simulink model "distmodel_v4"  (R2020b)
settings: Solver=FixedStepAuto  StartTime=0.0  StopTime=t_sim  FixedStep=TimeStep  RelTol=1e-3
values from neighbouring files (symbols this model uses):
  alt = 300    [main_disturbances.m]    (also in simple_propagator.m)
  D = [x_th-x_cog;y_th-y_cog;z_th-z_cog]/1e3    [momentumstorage.m]
  inc = rad2deg(inc)    [main_disturbances.m]    (also in simple_propagator.m)
  nu = rad2deg(nu)    [main_disturbances.m]    (also in simple_propagator.m)
  RAAN = rad2deg(RAAN)    [main_disturbances.m]    (also in simple_propagator.m)
  w = find(volume(:,y,z) == 1)    [calc_torque_v1.m]    (also in main_disturbances.m = rad2deg(w); simple_propagator.m = rad2deg(w))
undefined symbols (not defined in the file or in its folder): date, ecc, IonSataero, km, s, sat, SNAP_CONST_a3H0, SNAP_CONST_earth_mag_dipole, SNAP_magnets, SNAP_starting_ECI2ECEF_dcm
libraries: vrlib x15, dspmathops x8, sharedtransform x7, aerolibutil x5, simulink_extras x2, simulink x2, aerolibtransform2 x2, aerolibconvert2 x1, sharedutil x1, aerolibcelestial x1
settings Model: Creator=colpari  LastModifiedBy=colpari

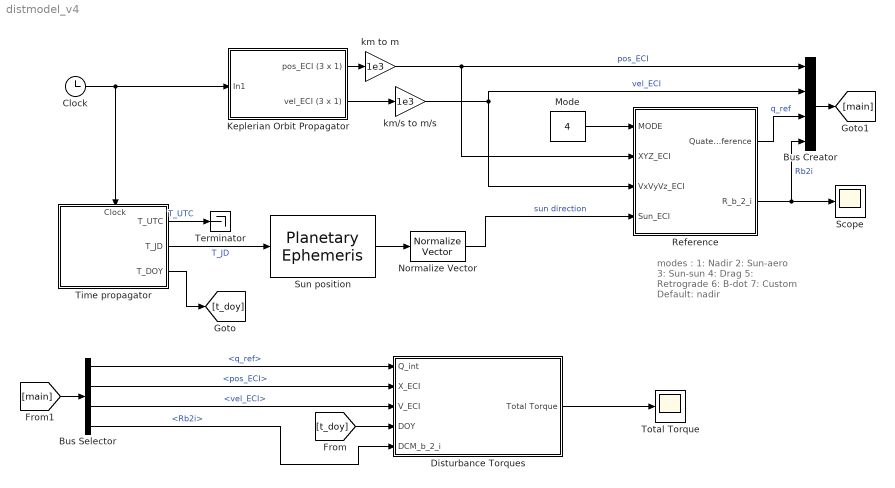
== system distmodel_v4 ==
  note: modes :
      | 1: Nadir
      | 2: Sun-aero
      | 3: Sun-sun
      | 4: Drag
      | 5: Retrograde
      | 6: B-dot
      | 7: Custom
      | Default: nadir
  Bus Creator : BusCreator  Inputs=4
  Bus Selector : BusSelector  OutputSignals=q_ref,pos_ECI,vel_ECI,Rb2i
  Clock : Clock
  "Disturbance Torques " : Subsystem
  Keplerian Orbit Propagator : Subsystem
  Mode : Constant  Value=4  OutDataTypeStr=int8
  Normalize Vector : vrlib/Utilities/Normalize Vector  maxzero=0
  Reference : Subsystem  TreatAsAtomicUnit=on
  Scope : Scope
  Sun position : aerolibcelestial/Planetary Ephemeris  kmflag=km,km/s  epochflag=Julian date  de=DE405  nCenter=Earth  nTarget=Sun  errorflag=Error  velflag=off
      settings: SourceProductBaseCode=AE
  Terminator : Terminator
  Time propagator : Subsystem
      settings: PortSchema="{\"entries\":[{\"content\":{\"sides\":[{\"content\":{\"connectorIds\":[]},\"type\":\"ConnectorPlacement.EquallySpacedRectSide\",\"uuid\":\"7ef5eb6e-74fd-40ed-a8ee-9d1a69b44829\"},{\"content\":{\"connectorIds\":[\"Out1\",\"Out2\",\"Out3\"],\"side\":\"RIGHT\"},\"type\":\"ConnectorPlacement.EquallySpacedRectSide\",\"uuid\":\"c2943143-c830-4f44-8257-0a7a59c653c3\"},{\"content\":{\"connectorIds\":[\"In1\"],\"side\":\"TOP\"},\"type\":\"ConnectorPlacement.EquallySpacedRectSide\",\"uuid\":\"75bbb385-8914-422a-90cf-596677817ce3\"},{\"content\":{\"connectorIds\":[],\"side\":\"HIDDEN\"},\"type\":\"ConnectorPlacement.EquallySpacedRectSide\",\"uuid\":\"39fbcd54-eaf8-409f-b881-9096903d4fff\"}]},\"type\":\"ConnectorPlacement.EquallySpacedConnector\",\"uuid\":\"f15d11f7-34b5-45ba-967f-26d924bb8ffd\"}],\"packageUris\":[\"http://schema.mathworks.com/mf0/Connector/R2020b\"],\"version\":\"1.0\"}"
  Total Torque : Scope
  km to m : Gain  Gain=1e3
  km/s to m/s : Gain  Gain=1e3
  wires:
  [t_doy] -> "Disturbance Torques "/4(DOY)
  "Disturbance Torques "/1("Total Torque ") -> Total Torque/1
  Bus Selector/3 -> "Disturbance Torques "/3(V_ECI)  "<vel_ECI>"
  Bus Selector/2 -> "Disturbance Torques "/2(X_ECI)  "<pos_ECI>"
  Clock/1 -> Keplerian Orbit Propagator/1(In1), Time propagator/1(Clock)
  Keplerian Orbit Propagator/1(pos_ECI (3 x 1)) -> km to m/1
  Keplerian Orbit Propagator/2(vel_ECI (3 x 1)) -> km/s to m/s/1
  Sun position/1 -> Normalize Vector/1
  Normalize Vector/1 -> Reference/4(Sun_ECI)  "sun direction"
  Time propagator/2(T_JD) -> Sun position/1  "T_JD"
  Reference/1(Quaternion Reference) -> Bus Creator/3  "q_ref"
  Time propagator/3(T_DOY) -> [t_doy]
  Bus Creator/1 -> [main]
  Time propagator/1(T_UTC) -> Terminator/1  "T_UTC"
  [main] -> Bus Selector/1
  km to m/1 -> Bus Creator/1, Reference/2(XYZ_ECI)  "pos_ECI"
  km/s to m/s/1 -> Bus Creator/2, Reference/3(VxVyVz_ECI)  "vel_ECI"
  Bus Selector/1 -> "Disturbance Torques "/1("Q_int ")  "<q_ref>"
  Reference/2(R_b_2_i) -> Bus Creator/4, Scope/1  "Rb2i"
  Bus Selector/4 -> "Disturbance Torques "/5(DCM_b_2_i)  "<Rb2i>"
  Mode/1 -> Reference/1(MODE)

== system distmodel_v4/Disturbance Torques  ==
  "Q_int " : Inport
  X_ECI : Inport  Port=2
  V_ECI : Inport  Port=3
  DOY : Inport  Port=4
  DCM_b_2_i : Inport  Port=5
  2 dist torques : Scope  NumInputPorts=2
  Add1 : Sum
  Aerodynamic Model : Subsystem
  Gravity Gradient Model : Subsystem
  Magnets : Subsystem  Commented=on
  Transpose1 : Math  Operator=transpose  SaturateOnIntegerOverflow=on
  "Total Torque " : Outport
  wires:
  Add1/1 -> "Total Torque "/1
  V_ECI/1 -> Aerodynamic Model/1(Velocity  (V) [m/s])
  X_ECI/1 -> Aerodynamic Model/2(Position (X) [m]), Gravity Gradient Model/1("Position (X) [m] ")
  Aerodynamic Model/2(Aero. Torque [N.m]1) -> 2 dist torques/1, Add1/1
  Gravity Gradient Model/1(Gravity Gradient [N.m]) -> 2 dist torques/2, Add1/2
  DCM_b_2_i/1 -> Transpose1/1
  Transpose1/1 -> Aerodynamic Model/3(Attitude (DCM_i2b)), Gravity Gradient Model/2(Attitude (DCMi2b))
  "Q_int "/1 -> Aerodynamic Model/4(Qref)

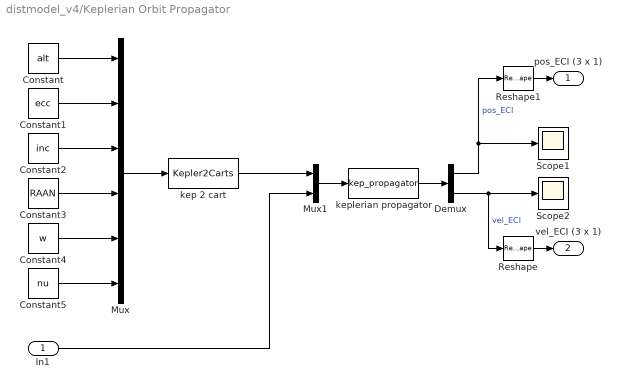
== system distmodel_v4/Keplerian Orbit Propagator ==
  In1 : Inport
  Constant : Constant  Value=alt
  Constant1 : Constant  Value=ecc
  Constant2 : Constant  Value=inc
  Constant3 : Constant  Value=RAAN
  Constant4 : Constant  Value=w
  Constant5 : Constant  Value=nu
  Demux : Demux  Outputs=2
  Mux : Mux  Inputs=6
  Mux1 : Mux  Inputs=2
  Reshape : Reshape  OutputDimensionality=Column vector (2-D)  OutputDimensions=[1,3]
  Reshape1 : Reshape  OutputDimensionality=Column vector (2-D)
  Scope1 : Scope
  Scope2 : Scope
  kep 2 cart : MATLABFcn  MATLABFcn=Kepler2Carts
  keplerian propagator : MATLABFcn  MATLABFcn=kep_propagator
  pos_ECI (3 x 1) : Outport
  vel_ECI (3 x 1) : Outport  Port=2
  wires:
  Mux/1 -> kep 2 cart/1
  Constant5/1 -> Mux/6
  Constant2/1 -> Mux/3
  kep 2 cart/1 -> Mux1/1
  Demux/2 -> Reshape/1, Scope2/1  "vel_ECI"
  Constant3/1 -> Mux/4
  Demux/1 -> Reshape1/1, Scope1/1  "pos_ECI"
  Constant4/1 -> Mux/5
  keplerian propagator/1 -> Demux/1
  Mux1/1 -> keplerian propagator/1
  Constant/1 -> Mux/1
  Constant1/1 -> Mux/2
  In1/1 -> Mux1/2
  Reshape/1 -> vel_ECI (3 x 1)/1
  Reshape1/1 -> pos_ECI (3 x 1)/1

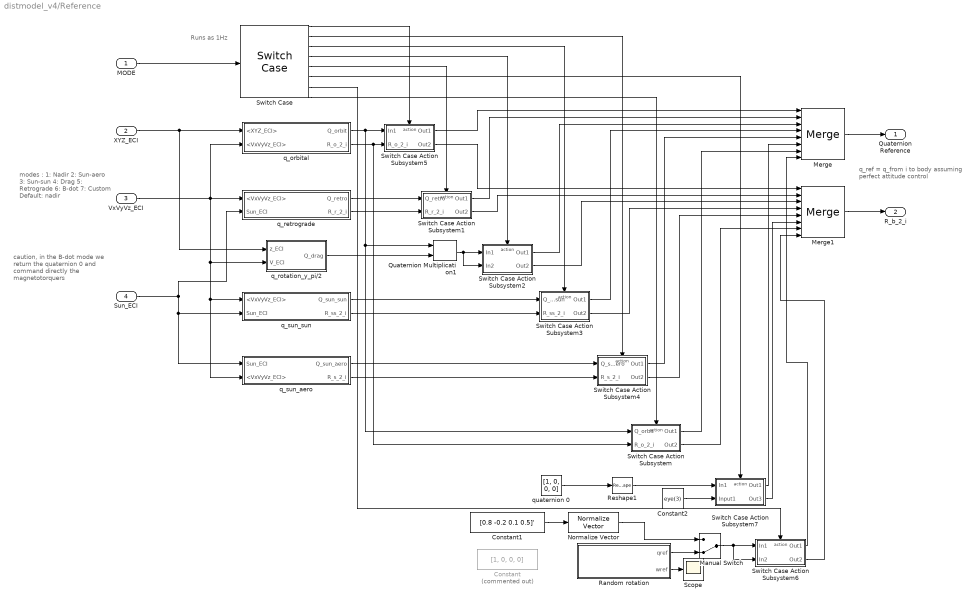
== system distmodel_v4/Reference ==
  note: caution, in the B-dot mode we return the quaternion 0 and command directly the magnetotorquers
  note: modes :
      | 1: Nadir
      | 2: Sun-aero
      | 3: Sun-sun
      | 4: Drag
      | 5: Retrograde
      | 6: B-dot
      | 7: Custom
      | Default: nadir
  note: Runs as 1Hz
  note: q_ref  = q_from i to body
      | assuming perfect attitude control
  MODE : Inport  OutMin=1  OutMax=100  OutDataTypeStr=int8
  XYZ_ECI : Inport  Port=2
  VxVyVz_ECI : Inport  Port=3
  Sun_ECI : Inport  Port=4
  Constant : Constant  Commented=on  Value=[1, 0, 0, 0]
  Constant1 : Constant  Value=[0.8 -0.2 0.1 0.5]'
  Constant2 : Constant  Value=eye(3)
  Manual Switch : ManualSwitch  CurrentSetting=0
  Merge : Merge  Inputs=8
  Merge1 : Merge  Inputs=8
  Normalize Vector : vrlib/Utilities/Normalize Vector  maxzero=0
  Quaternion Multiplication1 : aerolibutil/Quaternion Multiplication
  Random rotation : Subsystem
  Reshape1 : Reshape  OutputDimensionality=Column vector (2-D)
  Scope : Scope
  Switch Case : SwitchCase  CaseConditions={1, 2, 3, 4, 5, 6, 7}
  Switch Case Action Subsystem : Subsystem  TreatAsAtomicUnit=on
  Switch Case Action Subsystem1 : Subsystem  TreatAsAtomicUnit=on
  Switch Case Action Subsystem2 : Subsystem  TreatAsAtomicUnit=on
  Switch Case Action Subsystem3 : Subsystem  TreatAsAtomicUnit=on
  Switch Case Action Subsystem4 : Subsystem  TreatAsAtomicUnit=on
  Switch Case Action Subsystem5 : Subsystem  TreatAsAtomicUnit=on
  Switch Case Action Subsystem6 : Subsystem  TreatAsAtomicUnit=on
  Switch Case Action Subsystem7 : Subsystem  TreatAsAtomicUnit=on
  q_orbital : Subsystem
  q_retrograde : Subsystem
  q_rotation_y_pi/2 : Subsystem
  q_sun_aero : Subsystem
  q_sun_sun : Subsystem
  quaternion 0 : Constant  Value=[1, 0, 0, 0]
  Quaternion Reference : Outport  VectorParamsAs1DForOutWhenUnconnected=off
  R_b_2_i : Outport  Port=2
  wires:
  q_sun_sun/1(Q_sun_sun) -> Switch Case Action Subsystem3/1(Q_sun_sun)
  Sun_ECI/1 -> q_retrograde/2(Sun_ECI), q_sun_aero/1(Sun_ECI), q_sun_sun/2(Sun_ECI)
  MODE/1 -> Switch Case/1
  q_rotation_y_pi/2/1(Q_drag) -> Quaternion Multiplication1/2
  Switch Case/3 -> Switch Case Action Subsystem3/Action
  q_sun_aero/1(Q_sun_aero) -> Switch Case Action Subsystem4/1(Q_sun_aero)
  Merge/1 -> Quaternion Reference/1
  XYZ_ECI/1 -> q_orbital/1(<XYZ_ECI>), q_rotation_y_pi/2/1(z_ECI)
  Switch Case/5 -> Switch Case Action Subsystem1/Action
  Switch Case/4 -> Switch Case Action Subsystem2/Action
  quaternion 0/1 -> Reshape1/1
  VxVyVz_ECI/1 -> q_orbital/2(<VxVyVz_ECI>), q_retrograde/1(<VxVyVz_ECI>), q_sun_aero/2(<VxVyVz_ECI>), q_sun_sun/1(<VxVyVz_ECI>), q_rotation_y_pi/2/2(V_ECI)
  Switch Case/2 -> Switch Case Action Subsystem4/Action
  Quaternion Multiplication1/1 -> Switch Case Action Subsystem2/2(In2), Switch Case Action Subsystem2/1(In1)
  q_orbital/1(Q_orbit) -> Switch Case Action Subsystem5/1(In1), Quaternion Multiplication1/1, Switch Case Action Subsystem/1(Q_orbit)
  Switch Case/6 -> Switch Case Action Subsystem7/Action
  q_retrograde/1(Q_retro) -> Switch Case Action Subsystem1/1(Q_retro)
  Reshape1/1 -> Switch Case Action Subsystem7/1(In1)
  Merge1/1 -> R_b_2_i/1
  Switch Case Action Subsystem5/1(Out1) -> Merge/1
  Switch Case Action Subsystem5/2(Out2) -> Merge1/1
  Switch Case Action Subsystem1/1(Out1) -> Merge/2
  Switch Case Action Subsystem1/2(Out2) -> Merge1/2
  Switch Case Action Subsystem2/1(Out1) -> Merge/3
  Switch Case Action Subsystem2/2(Out2) -> Merge1/3
  Switch Case Action Subsystem3/1(Out1) -> Merge/4
  Switch Case Action Subsystem3/2(Out2) -> Merge1/4
  Switch Case Action Subsystem4/1(Out1) -> Merge/5
  Switch Case Action Subsystem4/2(Out2) -> Merge1/5
  Switch Case Action Subsystem/1(Out1) -> Merge/7
  Switch Case Action Subsystem/2(Out2) -> Merge1/7
  Switch Case Action Subsystem7/1(Out1) -> Merge/6
  Switch Case Action Subsystem7/2(Out3) -> Merge1/6
  Switch Case/1 -> Switch Case Action Subsystem5/Action
  Switch Case/8 -> Switch Case Action Subsystem/Action
  Switch Case/7 -> Switch Case Action Subsystem6/Action
  Switch Case Action Subsystem6/1(Out1) -> Merge/8
  Switch Case Action Subsystem6/2(Out2) -> Merge1/8
  Constant1/1 -> Normalize Vector/1
  Normalize Vector/1 -> Manual Switch/1
  Manual Switch/1 -> Switch Case Action Subsystem6/2(In2), Switch Case Action Subsystem6/1(In1)
  q_orbital/2(R_o_2_i) -> Switch Case Action Subsystem/2(R_o_2_i), Switch Case Action Subsystem5/2(R_o_2_i)
  q_sun_aero/2(R_s_2_i) -> Switch Case Action Subsystem4/2(R_s_2_i)
  q_sun_sun/2(R_ss_2_i) -> Switch Case Action Subsystem3/2(R_ss_2_i)
  q_retrograde/2(R_r_2_i) -> Switch Case Action Subsystem1/2(R_r_2_i)
  Constant2/1 -> Switch Case Action Subsystem7/2(Input1)
  Random rotation/1(qref) -> Manual Switch/2
  Random rotation/2(wref) -> Scope/1

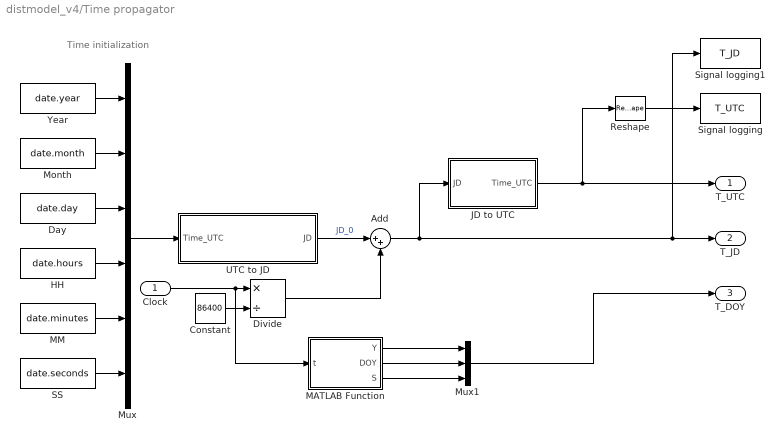
== system distmodel_v4/Time propagator ==
  note: Time initialization
  Clock : Inport
  Add : Sum  Inputs=|++
  Constant : Constant  Value=86400
  Day : Constant  Value=date.day
  Divide : Product  Inputs=*/
  HH : Constant  Value=date.hours
  JD to UTC : MATLAB Function  TreatAsAtomicUnit=on
  MATLAB Function : MATLAB Function  TreatAsAtomicUnit=on
  MM : Constant  Value=date.minutes
  Month : Constant  Value=date.month
  Mux : Mux  Inputs=6
  Mux1 : Mux  Inputs=3
  Reshape : Reshape
  SS : Constant  Value=date.seconds
  Signal logging : ToWorkspace  VariableName=T_UTC  SaveFormat=Timeseries  SampleTime=1
      settings: Save2DSignal=2-D array (concatenate along first dimension)
  Signal logging1 : ToWorkspace  VariableName=T_JD  SaveFormat=Timeseries  SampleTime=1
      settings: Save2DSignal=2-D array (concatenate along first dimension)
  UTC to JD : MATLAB Function  TreatAsAtomicUnit=on
  Year : Constant  Value=date.year
  T_UTC : Outport  VectorParamsAs1DForOutWhenUnconnected=off
  T_JD : Outport  Port=2  VectorParamsAs1DForOutWhenUnconnected=off
  T_DOY : Outport  Port=3
  wires:
  UTC to JD/1(JD) -> Add/1  "JD_0"
  Clock/1 -> MATLAB Function/1(t), Divide/1
  Constant/1 -> Divide/2
  JD to UTC/1(Time_UTC) -> T_UTC/1, Reshape/1
  Divide/1 -> Add/2
  Mux/1 -> UTC to JD/1(Time_UTC)
  Day/1 -> Mux/3
  Month/1 -> Mux/2
  Year/1 -> Mux/1
  HH/1 -> Mux/4
  MM/1 -> Mux/5
  SS/1 -> Mux/6
  Reshape/1 -> Signal logging/1
  Add/1 -> Signal logging1/1, T_JD/1, JD to UTC/1(JD)
  MATLAB Function/1(Y) -> Mux1/1
  MATLAB Function/2(DOY) -> Mux1/2
  MATLAB Function/3(S) -> Mux1/3
  Mux1/1 -> T_DOY/1

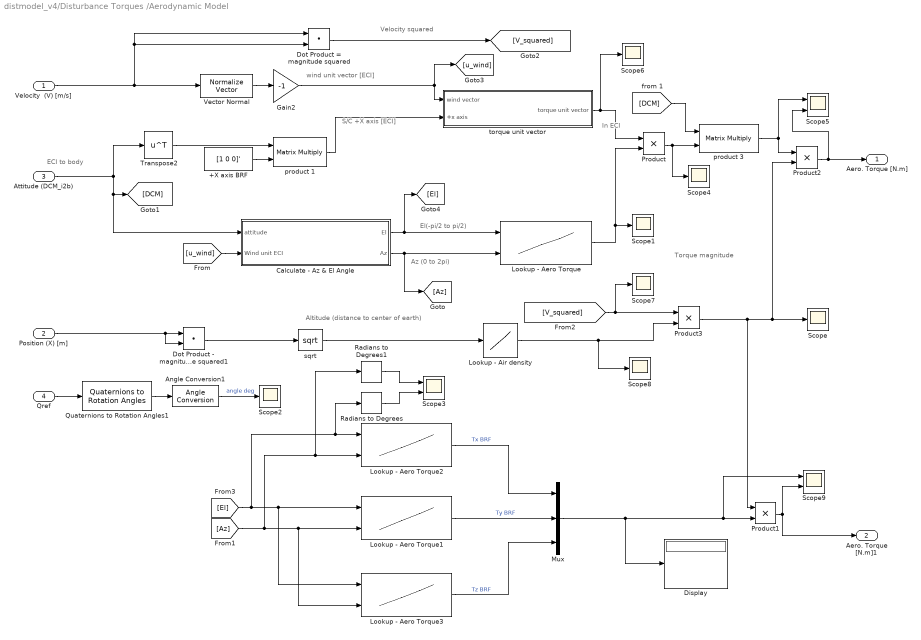
== system distmodel_v4/Disturbance Torques /Aerodynamic Model ==
  note: Az (0 to 2pi)
  note: wind unit vector [ECI]
  note: Torque magnitude
  note: S/C +X axis [ECI]
  note: In ECI
  note: ECI to body
  note: Velocity squared
  note: El(-pi/2 to pi/2)
  note: Altitude (distance to center of earth)
  Velocity  (V) [m/s] : Inport
  Position (X) [m] : Inport  Port=2
  Attitude (DCM_i2b) : Inport  Port=3
  Qref : Inport  Port=4
  +X axis BRF : Constant  Value=[1 0 0]'
  Angle Conversion1 : aerolibconvert2/Angle Conversion  IU=rad  OU=deg
  Calculate - Az & El Angle : Subsystem
  Display : Display
  Dot Product - magnitude squared1 : DotProduct  InputSameDT=on  OutDataTypeStr=Inherit: Inherit via internal rule
  Dot Product = magnitude squared : DotProduct  InputSameDT=on  OutDataTypeStr=Inherit: Inherit via internal rule
  Gain2 : Gain  Gain=-1
  Lookup - Aero Torque : Lookup2D  RowIndex=IonSataero.Az  ColumnIndex=IonSataero.El  Table=IonSataero.T
  Lookup - Aero Torque1 : Lookup2D  RowIndex=IonSataero.Az  ColumnIndex=IonSataero.El  Table=IonSataero.Ty
  Lookup - Aero Torque2 : Lookup2D  RowIndex=IonSataero.Az  ColumnIndex=IonSataero.El  Table=IonSataero.Tx
  Lookup - Aero Torque3 : Lookup2D  RowIndex=IonSataero.Az  ColumnIndex=IonSataero.El  Table=IonSataero.Tz
  Lookup - Air density : Lookup  InputValues=IonSataero.alt_range*1000 + 6378100  Table=IonSataero.av_density_vs_alt
  Mux : Mux  Inputs=3
  Product{,1..3} (4 alike) : Product  RndMeth=Zero
  Quaternions to Rotation Angles1 : sharedtransform/Quaternions to Rotation Angles  rotationOrder=ZYX  aMode=aMode
      settings: SourceProductBaseCode=AE,PW,MT,UV,VE,VP
  Radians to Degrees : simulink_extras/Transformations/Radians to Degrees
  Radians to Degrees1 : simulink_extras/Transformations/Radians to Degrees
  Scope{,1..2,4,6..8} (7 alike) : Scope
  Scope3 : Scope  NumInputPorts=2
  Scope5 : Scope  NumInputPorts=2
  Scope9 : Scope  NumInputPorts=2
  Transpose2 : Math  Operator=transpose  SignedPower=on  SaturateOnIntegerOverflow=on
  Vector Normal : vrlib/Utilities/Normalize Vector  maxzero=0
  product 1 : Product  Multiplication=Matrix(*)  RndMeth=Zero
  product 3 : Product  Multiplication=Matrix(*)  RndMeth=Zero
  sqrt : Math  Operator=sqrt  SignedPower=on  SaturateOnIntegerOverflow=on
  torque unit vector : Subsystem
  Aero. Torque [N.m] : Outport
  Aero. Torque [N.m]1 : Outport  Port=2
  wires:
  Dot Product = magnitude squared/1 -> [V_squared]
  Vector Normal/1 -> Gain2/1
  Gain2/1 -> [u_wind], torque unit vector/1(wind vector)
  product 1/1 -> torque unit vector/2(+x axis)
  torque unit vector/1(torque unit vector) -> Scope6/1, Product/1
  Lookup - Aero Torque/1 -> Scope1/1, Product/2
  [DCM] -> product 3/1
  +X axis BRF/1 -> product 1/2
  Product/1 -> Scope4/1, product 3/2
  Transpose2/1 -> product 1/1
  Attitude (DCM_i2b)/1 -> Calculate - Az & El Angle/1(attitude), [DCM], Transpose2/1
  Position (X) [m]/1 -> Dot Product - magnitude squared1/1, Dot Product - magnitude squared1/2
  Dot Product - magnitude squared1/1 -> sqrt/1
  sqrt/1 -> Lookup - Air density/1
  Lookup - Air density/1 -> Scope8/1, Product3/2
  [V_squared] -> Scope7/1, Product3/1
  Product2/1 -> Scope5/2, Aero. Torque [N.m]/1
  product 3/1 -> Scope5/1, Product2/1
  Velocity  (V) [m/s]/1 -> Vector Normal/1, Dot Product = magnitude squared/2, Dot Product = magnitude squared/1
  Radians to Degrees1/1 -> Scope3/1
  Radians to Degrees/1 -> Scope3/2
  Qref/1 -> Quaternions to Rotation Angles1/1
  Quaternions to Rotation Angles1/1 -> Angle Conversion1/1
  Angle Conversion1/1 -> Scope2/1  "angle deg"
  [u_wind] -> Calculate - Az & El Angle/2(Wind unit ECI)
  Calculate - Az & El Angle/2(Az) -> [Az], Lookup - Aero Torque/2
  Calculate - Az & El Angle/1(El) -> [El], Lookup - Aero Torque/1
  [El] -> Radians to Degrees/1, Lookup - Aero Torque2/1, Lookup - Aero Torque3/1, Lookup - Aero Torque1/1
  [Az] -> Radians to Degrees1/1, Lookup - Aero Torque2/2, Lookup - Aero Torque3/2, Lookup - Aero Torque1/2
  Lookup - Aero Torque1/1 -> Mux/2  "Ty BRF"
  Lookup - Aero Torque2/1 -> Mux/1  "Tx BRF"
  Lookup - Aero Torque3/1 -> Mux/3  "Tz BRF"
  Mux/1 -> Display/1, Product1/2, Scope9/1
  Product3/1 -> Product1/1, Scope/1, Product2/2
  Product1/1 -> Aero. Torque [N.m]1/1, Scope9/2

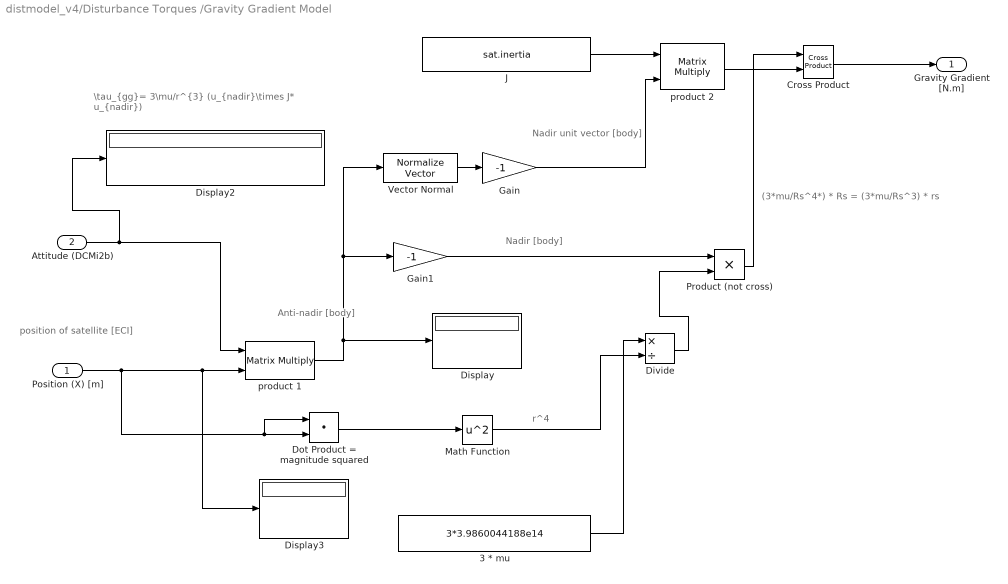
== system distmodel_v4/Disturbance Torques /Gravity Gradient Model ==
  note: \tau_{gg}= 3\mu/r^{3} (u_{nadir}\times J* u_{nadir})
  note: (3*mu/Rs^4*) * Rs = (3*mu/Rs^3) * rs
  note: Nadir [body]
  note: position of satellite [ECI]
  note: Nadir unit vector
      | [body]
  note: Anti-nadir [body]
  note: r^4
  "Position (X) [m] " : Inport
  Attitude (DCMi2b) : Inport  Port=2
  3 * mu : Constant  Value=3*3.9860044188e14
  Cross Product : vrlib/Utilities/Cross Product
  Display : Display
  Display2 : Display
  Display3 : Display
  Divide : Product  Inputs=*/
  Dot Product = magnitude squared : DotProduct  InputSameDT=on  OutDataTypeStr=Inherit: Inherit via internal rule
  Gain : Gain  Gain=-1
  Gain1 : Gain  Gain=-1
  J : Constant  Value=sat.inertia
  Math Function : Math  Operator=square  SignedPower=on  SaturateOnIntegerOverflow=on
  Product (not cross) : Product  RndMeth=Zero
  Vector Normal : vrlib/Utilities/Normalize Vector  maxzero=0
  product 1 : Product  Multiplication=Matrix(*)  RndMeth=Zero
  product 2 : Product  Multiplication=Matrix(*)  RndMeth=Zero
  Gravity Gradient [N.m] : Outport
  wires:
  Product (not cross)/1 -> Cross Product/1
  Divide/1 -> Product (not cross)/2
  3 * mu/1 -> Divide/1
  Math Function/1 -> Divide/2
  Vector Normal/1 -> Gain/1
  Cross Product/1 -> Gravity Gradient [N.m]/1
  Dot Product = magnitude squared/1 -> Math Function/1
  Gain/1 -> product 2/2
  product 2/1 -> Cross Product/2
  J/1 -> product 2/1
  Attitude (DCMi2b)/1 -> Display2/1, product 1/1
  product 1/1 -> Vector Normal/1, Gain1/1, Display/1
  Gain1/1 -> Product (not cross)/1
  "Position (X) [m] "/1 -> product 1/2, Display3/1, Dot Product = magnitude squared/2, Dot Product = magnitude squared/1

== system distmodel_v4/Disturbance Torques /Magnets ==
  note: T = m X B
  note: B_earth [body]
  note: ECI to Body
  Position (X) : Inport
  Attitude (DCM) : Inport  Port=2
  Cross Product : vrlib/Utilities/Cross Product
  Eearth L-Shell Magnetic Model : Subsystem
  Product : Product  Multiplication=Matrix(*)  RndMeth=Zero
  Transpose : Math  Operator=transpose  SignedPower=on  SaturateOnIntegerOverflow=on
  constant : Constant  Value=SNAP_magnets
  MagneticTorque (N.m) : Outport
  B (Tesla) [ECI] : Outport  Port=2
  wires:
  Position (X)/1 -> Eearth L-Shell Magnetic Model/1(Position in ECI)
  Product/1 -> Cross Product/2
  Cross Product/1 -> MagneticTorque (N.m)/1
  constant/1 -> Cross Product/1
  Attitude (DCM)/1 -> Product/1
  Eearth L-Shell Magnetic Model/1(B (Tesla) in ECI) -> Transpose/1, B (Tesla) [ECI]/1
  Transpose/1 -> Product/2

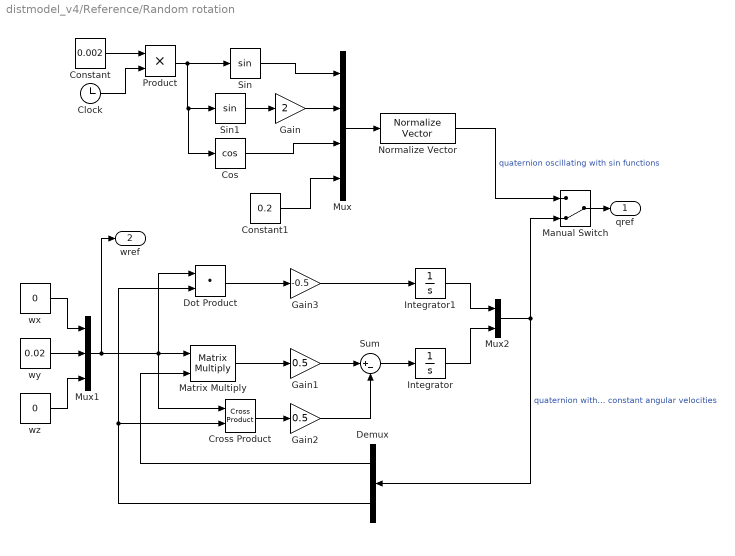
== system distmodel_v4/Reference/Random rotation ==
  Clock : Clock
      settings: Decimation=TimeStep
  Constant : Constant  Value=0.002
  Constant1 : Constant  Value=0.2
  Cos : Trigonometry  Operator=cos
  Cross Product : vrlib/Utilities/Cross Product
  Demux : Demux  Outputs=[1;3]
  Dot Product : DotProduct  InputSameDT=on  OutDataTypeStr=Inherit: Inherit via internal rule
  Gain : Gain  Gain=2
  Gain1 : Gain  Gain=0.5
  Gain2 : Gain  Gain=0.5
  Gain3 : Gain  Gain=-0.5
  Integrator : Integrator  InitialCondition=[0;0;0]
  Integrator1 : Integrator  InitialCondition=1
  Manual Switch : ManualSwitch  CurrentSetting=0
  Matrix Multiply : Product  Multiplication=Matrix(*)
  Mux : Mux
  Mux1 : Mux  Inputs=3
  Mux2 : Mux  Inputs=[1;3]
  Normalize Vector : vrlib/Utilities/Normalize Vector  maxzero=0
  Product : Product
  Sin : Trigonometry
  Sin1 : Trigonometry
  Sum : Sum  Inputs=|+-
  wx : Constant  Value=0
  wy : Constant  Value=0.02
  wz : Constant  Value=0
  qref : Outport
  wref : Outport  Port=2
  wires:
  Mux/1 -> Normalize Vector/1
  Normalize Vector/1 -> Manual Switch/1  "quaternion oscillating with sin functions"
  Constant/1 -> Product/1
  Clock/1 -> Product/2
  Product/1 -> Cos/1, Sin1/1, Sin/1
  Sin/1 -> Mux/1
  Sin1/1 -> Gain/1
  Gain/1 -> Mux/2
  Cos/1 -> Mux/3
  Constant1/1 -> Mux/4
  Manual Switch/1 -> qref/1
  wx/1 -> Mux1/1
  wy/1 -> Mux1/2
  wz/1 -> Mux1/3
  Mux1/1 -> wref/1, Dot Product/1, Cross Product/1, Matrix Multiply/1
  Matrix Multiply/1 -> Gain1/1
  Gain1/1 -> Sum/1
  Sum/1 -> Integrator/1
  Integrator/1 -> Mux2/2
  Mux2/1 -> Demux/1, Manual Switch/2  "quaternion with constant angular velocities"
  Demux/1 -> Matrix Multiply/2
  Cross Product/1 -> Gain2/1
  Gain2/1 -> Sum/2
  Dot Product/1 -> Gain3/1
  Gain3/1 -> Integrator1/1
  Integrator1/1 -> Mux2/1
  Demux/2 -> Cross Product/2, Dot Product/2

== system distmodel_v4/Reference/Switch Case Action Subsystem ==
  Q_orbit : Inport
  R_o_2_i : Inport  Port=2
  Action Port : ActionPort  ActionPortLabel=default:
  Out1 : Outport  VectorParamsAs1DForOutWhenUnconnected=off
  Out2 : Outport  Port=2  VectorParamsAs1DForOutWhenUnconnected=off
  wires:
  Q_orbit/1 -> Out1/1
  R_o_2_i/1 -> Out2/1

== system distmodel_v4/Reference/Switch Case Action Subsystem1 ==
  Q_retro : Inport
  R_r_2_i : Inport  Port=2
  Action Port : ActionPort  ActionPortLabel=case [ 5 ]:
  Out1 : Outport  VectorParamsAs1DForOutWhenUnconnected=off
  Out2 : Outport  Port=2  VectorParamsAs1DForOutWhenUnconnected=off
  wires:
  Q_retro/1 -> Out1/1
  R_r_2_i/1 -> Out2/1

== system distmodel_v4/Reference/Switch Case Action Subsystem2 ==
  In1 : Inport
  In2 : Inport  Port=2
  Action Port : ActionPort  ActionPortLabel=case [ 4 ]:
  Quaternions to Direction Cosine Matrix : sharedtransform/Quaternions to  Direction Cosine Matrix  aMode=aMode
      settings: SourceProductBaseCode=AE,PW,MT,UV,VE,VP
  Out1 : Outport  VectorParamsAs1DForOutWhenUnconnected=off
  Out2 : Outport  Port=2  VectorParamsAs1DForOutWhenUnconnected=off
  wires:
  In1/1 -> Out1/1
  In2/1 -> Quaternions to Direction Cosine Matrix/1
  Quaternions to Direction Cosine Matrix/1 -> Out2/1

== system distmodel_v4/Reference/Switch Case Action Subsystem3 ==
  Q_sun_sun : Inport
  R_ss_2_i : Inport  Port=2
  Action Port : ActionPort  ActionPortLabel=case [ 3 ]:
  Out1 : Outport  VectorParamsAs1DForOutWhenUnconnected=off
  Out2 : Outport  Port=2  VectorParamsAs1DForOutWhenUnconnected=off
  wires:
  Q_sun_sun/1 -> Out1/1
  R_ss_2_i/1 -> Out2/1

== system distmodel_v4/Reference/Switch Case Action Subsystem4 ==
  Q_sun_aero : Inport
  R_s_2_i : Inport  Port=2
  Action Port : ActionPort  ActionPortLabel=case [ 2 ]:
  Out1 : Outport  VectorParamsAs1DForOutWhenUnconnected=off
  Out2 : Outport  Port=2  VectorParamsAs1DForOutWhenUnconnected=off
  wires:
  Q_sun_aero/1 -> Out1/1
  R_s_2_i/1 -> Out2/1

== system distmodel_v4/Reference/Switch Case Action Subsystem5 ==
  In1 : Inport
  R_o_2_i : Inport  Port=2
  Action Port : ActionPort  ActionPortLabel=case [ 1 ]:
  Out1 : Outport  VectorParamsAs1DForOutWhenUnconnected=off
  Out2 : Outport  Port=2  VectorParamsAs1DForOutWhenUnconnected=off
  wires:
  In1/1 -> Out1/1
  R_o_2_i/1 -> Out2/1

== system distmodel_v4/Reference/Switch Case Action Subsystem6 ==
  In1 : Inport
  In2 : Inport  Port=2
  Action Port : ActionPort  ActionPortLabel=case [ 7 ]:
  Quaternions to Direction Cosine Matrix : sharedtransform/Quaternions to  Direction Cosine Matrix  aMode=aMode
      settings: SourceProductBaseCode=AE,PW,MT,UV,VE,VP
  Out1 : Outport  VectorParamsAs1DForOutWhenUnconnected=off
  Out2 : Outport  Port=2  VectorParamsAs1DForOutWhenUnconnected=off
  wires:
  In1/1 -> Out1/1
  In2/1 -> Quaternions to Direction Cosine Matrix/1
  Quaternions to Direction Cosine Matrix/1 -> Out2/1

== system distmodel_v4/Reference/Switch Case Action Subsystem7 ==
  In1 : Inport
  Input1 : Inport  Port=2
  Action Port : ActionPort  ActionPortLabel=case [ 6 ]:
  Out1 : Outport  VectorParamsAs1DForOutWhenUnconnected=off
  Out3 : Outport  Port=2  VectorParamsAs1DForOutWhenUnconnected=off
  wires:
  In1/1 -> Out1/1
  Input1/1 -> Out3/1

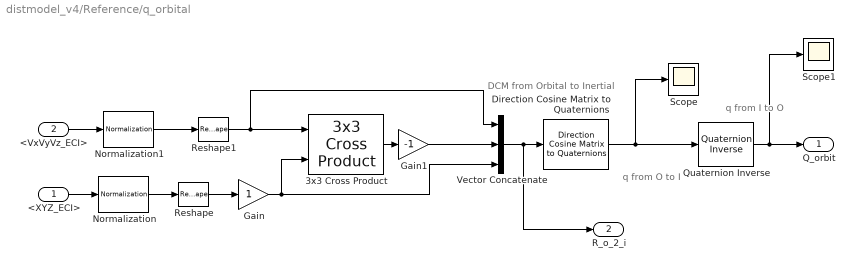
== system distmodel_v4/Reference/q_orbital ==
  note: DCM from Orbital to Inertial
  note: q from O to I
  note: q from I to O
  <XYZ_ECI> : Inport
  <VxVyVz_ECI> : Inport  Port=2
  3x3 Cross Product : sharedutil/3x3 Cross Product  aMode=aMode
      settings: SourceProductBaseCode=AE,PW,MT,UV,VE,VP
  Direction Cosine Matrix to Quaternions : sharedtransform/Direction Cosine Matrix  to Quaternions  aMode=0  action=None  tolerance=eps(2)
      settings: SourceProductBaseCode=AE,PW,MT,UV,VE,VP
  Gain : Gain
  Gain1 : Gain  Gain=-1
  Normalization : dspmathops/Normalization  NormType=2-norm  Bias=1e-10  NormOver=Each column  Dimension=1  roundingMode=Floor  overflowMode=off  accumDataTypeStr=Inherit: Same as product output  accumLastDataTypeStr=Inherit: Same as product output  outputDataTypeStr=Inherit: Same as product output  outputMin=[]  outputMax=[]  outputLastDataTypeStr=Inherit: Same as product output
  Normalization1 : dspmathops/Normalization  NormType=2-norm  Bias=1e-10  NormOver=Each column  Dimension=1  roundingMode=Floor  overflowMode=off  accumDataTypeStr=Inherit: Same as product output  accumLastDataTypeStr=Inherit: Same as product output  outputDataTypeStr=Inherit: Same as product output  outputMin=[]  outputMax=[]  outputLastDataTypeStr=Inherit: Same as product output
  Quaternion Inverse : aerolibutil/Quaternion Inverse
  Reshape : Reshape  OutputDimensionality=Column vector (2-D)
  Reshape1 : Reshape  OutputDimensionality=Column vector (2-D)
  Scope : Scope
  Scope1 : Scope
  Vector Concatenate : Concatenate  NumInputs=3  Mode=Multidimensional array  ConcatenateDimension=2
  Q_orbit : Outport  VectorParamsAs1DForOutWhenUnconnected=off
  R_o_2_i : Outport  Port=2  VectorParamsAs1DForOutWhenUnconnected=off
  wires:
  Normalization/1 -> Reshape/1
  Normalization1/1 -> Reshape1/1
  <VxVyVz_ECI>/1 -> Normalization1/1
  Reshape1/1 -> 3x3 Cross Product/1, Vector Concatenate/1
  <XYZ_ECI>/1 -> Normalization/1
  Reshape/1 -> Gain/1
  Gain/1 -> 3x3 Cross Product/2, Vector Concatenate/3
  Direction Cosine Matrix to Quaternions/1 -> Scope/1, Quaternion Inverse/1
  3x3 Cross Product/1 -> Gain1/1
  Gain1/1 -> Vector Concatenate/2
  Vector Concatenate/1 -> R_o_2_i/1, Direction Cosine Matrix to Quaternions/1
  Quaternion Inverse/1 -> Scope1/1, Q_orbit/1

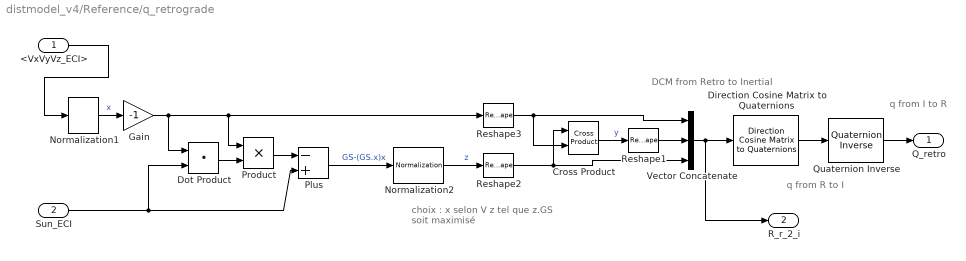
== system distmodel_v4/Reference/q_retrograde ==
  note: q from I to R
  note: q from R to I
  note: DCM from Retro to Inertial
  note: choix :
      | x selon V
      | z tel que z.GS soit maximisé
  <VxVyVz_ECI> : Inport
  Sun_ECI : Inport  Port=2
  Cross Product : vrlib/Utilities/Cross Product
  Direction Cosine Matrix to Quaternions : sharedtransform/Direction Cosine Matrix  to Quaternions  aMode=0  action=None  tolerance=eps(2)
      settings: SourceProductBaseCode=AE,PW,MT,UV,VE,VP
  Dot Product : DotProduct  InputSameDT=on  OutDataTypeStr=Inherit: Inherit via internal rule
  Gain : Gain  Gain=-1
  Normalization1 : dspmathops/Normalization  NormType=2-norm  Bias=1e-10  NormOver=Each column  Dimension=1  roundingMode=Floor  overflowMode=off  accumDataTypeStr=Inherit: Same as product output  accumLastDataTypeStr=Inherit: Same as product output  outputDataTypeStr=Inherit: Same as product output  outputMin=[]  outputMax=[]  outputLastDataTypeStr=Inherit: Same as product output
  Normalization2 : dspmathops/Normalization  NormType=2-norm  Bias=1e-10  NormOver=Each column  Dimension=1  roundingMode=Floor  overflowMode=off  accumDataTypeStr=Inherit: Same as product output  accumLastDataTypeStr=Inherit: Same as product output  outputDataTypeStr=Inherit: Same as product output  outputMin=[]  outputMax=[]  outputLastDataTypeStr=Inherit: Same as product output
  Plus : Sum  Inputs=-+
  Product : Product
  Quaternion Inverse : aerolibutil/Quaternion Inverse
  Reshape1 : Reshape  OutputDimensionality=Column vector (2-D)
  Reshape2 : Reshape  OutputDimensionality=Column vector (2-D)
  Reshape3 : Reshape  OutputDimensionality=Column vector (2-D)
  Vector Concatenate : Concatenate  NumInputs=3  Mode=Multidimensional array  ConcatenateDimension=2
  Q_retro : Outport  VectorParamsAs1DForOutWhenUnconnected=off
  R_r_2_i : Outport  Port=2  VectorParamsAs1DForOutWhenUnconnected=off
  wires:
  Quaternion Inverse/1 -> Q_retro/1
  Reshape2/1 -> Vector Concatenate/3, Cross Product/1
  Reshape3/1 -> Vector Concatenate/1, Cross Product/2
  Product/1 -> Plus/1
  Dot Product/1 -> Product/2
  Cross Product/1 -> Reshape1/1  "y"
  Normalization2/1 -> Reshape2/1  "z"
  Plus/1 -> Normalization2/1  "GS-(GS.x)x"
  Sun_ECI/1 -> Dot Product/2, Plus/2
  Vector Concatenate/1 -> R_r_2_i/1, Direction Cosine Matrix to Quaternions/1
  Direction Cosine Matrix to Quaternions/1 -> Quaternion Inverse/1
  Normalization1/1 -> Gain/1  "x"
  <VxVyVz_ECI>/1 -> Normalization1/1
  Reshape1/1 -> Vector Concatenate/2
  Gain/1 -> Dot Product/1, Product/1, Reshape3/1

== system distmodel_v4/Reference/q_rotation_y_pi//2 ==
  z_ECI : Inport
  V_ECI : Inport  Port=2
  Cross Product : vrlib/Utilities/Cross Product
  Product : Product
  Reshape1 : Reshape  OutputDimensionality=Column vector (2-D)
  Vector Concatenate1 : Concatenate  Mode=Multidimensional array
  cos pi/4 : Constant  Value=[sqrt(2)]
  sin pi/4 : Constant  Value=sqrt(2)
  Q_drag : Outport  VectorParamsAs1DForOutWhenUnconnected=off
  wires:
  cos pi/4/1 -> Vector Concatenate1/1
  Vector Concatenate1/1 -> Q_drag/1
  sin pi/4/1 -> Product/2
  z_ECI/1 -> Cross Product/1
  V_ECI/1 -> Cross Product/2
  Cross Product/1 -> Product/1  "y"
  Reshape1/1 -> Vector Concatenate1/2
  Product/1 -> Reshape1/1

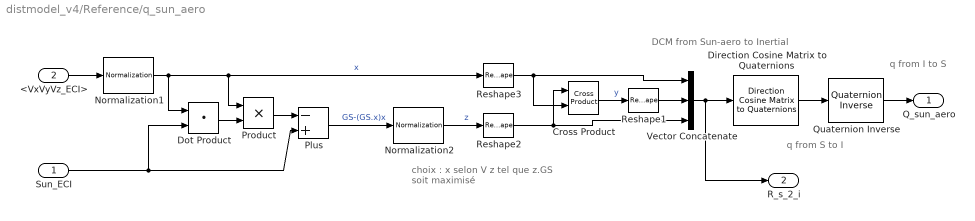
== system distmodel_v4/Reference/q_sun_aero ==
  note: q from I to S
  note: q from S to I
  note: DCM from Sun-aero to Inertial
  note: choix :
      | x selon V
      | z tel que z.GS soit maximisé
  Sun_ECI : Inport
  <VxVyVz_ECI> : Inport  Port=2
  Cross Product : vrlib/Utilities/Cross Product
  Direction Cosine Matrix to Quaternions : sharedtransform/Direction Cosine Matrix  to Quaternions  aMode=0  action=None  tolerance=eps(2)
      settings: SourceProductBaseCode=AE,PW,MT,UV,VE,VP
  Dot Product : DotProduct  InputSameDT=on  OutDataTypeStr=Inherit: Inherit via internal rule
  Normalization1 : dspmathops/Normalization  NormType=2-norm  Bias=1e-10  NormOver=Each column  Dimension=1  roundingMode=Floor  overflowMode=off  accumDataTypeStr=Inherit: Same as product output  accumLastDataTypeStr=Inherit: Same as product output  outputDataTypeStr=Inherit: Same as product output  outputMin=[]  outputMax=[]  outputLastDataTypeStr=Inherit: Same as product output
  Normalization2 : dspmathops/Normalization  NormType=2-norm  Bias=1e-10  NormOver=Each column  Dimension=1  roundingMode=Floor  overflowMode=off  accumDataTypeStr=Inherit: Same as product output  accumLastDataTypeStr=Inherit: Same as product output  outputDataTypeStr=Inherit: Same as product output  outputMin=[]  outputMax=[]  outputLastDataTypeStr=Inherit: Same as product output
  Plus : Sum  Inputs=-+
  Product : Product
  Quaternion Inverse : aerolibutil/Quaternion Inverse
  Reshape1 : Reshape  OutputDimensionality=Column vector (2-D)
  Reshape2 : Reshape  OutputDimensionality=Column vector (2-D)
  Reshape3 : Reshape  OutputDimensionality=Column vector (2-D)
  Vector Concatenate : Concatenate  NumInputs=3  Mode=Multidimensional array  ConcatenateDimension=2
  Q_sun_aero : Outport  VectorParamsAs1DForOutWhenUnconnected=off
  R_s_2_i : Outport  Port=2  VectorParamsAs1DForOutWhenUnconnected=off
  wires:
  Quaternion Inverse/1 -> Q_sun_aero/1
  Reshape2/1 -> Vector Concatenate/3, Cross Product/1
  Reshape3/1 -> Vector Concatenate/1, Cross Product/2
  Product/1 -> Plus/1
  Dot Product/1 -> Product/2
  Cross Product/1 -> Reshape1/1  "y"
  Normalization2/1 -> Reshape2/1  "z"
  Plus/1 -> Normalization2/1  "GS-(GS.x)x"
  Sun_ECI/1 -> Dot Product/2, Plus/2
  Vector Concatenate/1 -> R_s_2_i/1, Direction Cosine Matrix to Quaternions/1
  Direction Cosine Matrix to Quaternions/1 -> Quaternion Inverse/1
  Normalization1/1 -> Dot Product/1, Product/1, Reshape3/1  "x"
  <VxVyVz_ECI>/1 -> Normalization1/1
  Reshape1/1 -> Vector Concatenate/2

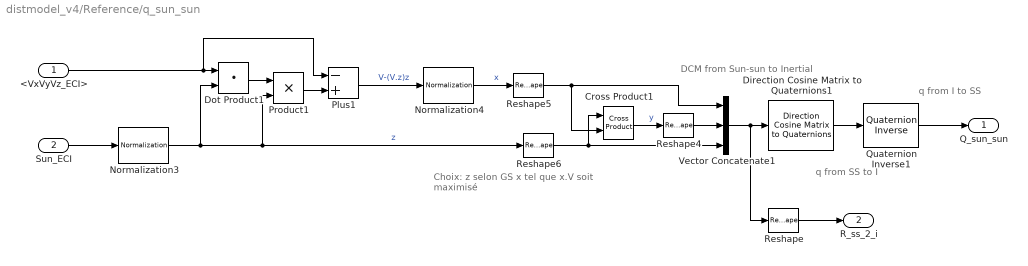
== system distmodel_v4/Reference/q_sun_sun ==
  note: Choix:
      | z selon GS
      | x tel que x.V soit maximisé
  note: DCM from Sun-sun to Inertial
  note: q from I to SS
  note: q from SS to I
  <VxVyVz_ECI> : Inport
  Sun_ECI : Inport  Port=2
  Cross Product1 : vrlib/Utilities/Cross Product
  Direction Cosine Matrix to Quaternions1 : sharedtransform/Direction Cosine Matrix  to Quaternions  aMode=0  action=None  tolerance=eps(2)
      settings: SourceProductBaseCode=AE,PW,MT,UV,VE,VP
  Dot Product1 : DotProduct  InputSameDT=on  OutDataTypeStr=Inherit: Inherit via internal rule
  Normalization3 : dspmathops/Normalization  NormType=2-norm  Bias=1e-10  NormOver=Each column  Dimension=1  roundingMode=Floor  overflowMode=off  accumDataTypeStr=Inherit: Same as product output  accumLastDataTypeStr=Inherit: Same as product output  outputDataTypeStr=Inherit: Same as product output  outputMin=[]  outputMax=[]  outputLastDataTypeStr=Inherit: Same as product output
  Normalization4 : dspmathops/Normalization  NormType=2-norm  Bias=1e-10  NormOver=Each column  Dimension=1  roundingMode=Floor  overflowMode=off  accumDataTypeStr=Inherit: Same as product output  accumLastDataTypeStr=Inherit: Same as product output  outputDataTypeStr=Inherit: Same as product output  outputMin=[]  outputMax=[]  outputLastDataTypeStr=Inherit: Same as product output
  Plus1 : Sum  Inputs=-+
  Product1 : Product
  Quaternion Inverse1 : aerolibutil/Quaternion Inverse
  Reshape : Reshape  OutputDimensionality=Customize  OutputDimensions=[3,3]
  Reshape4 : Reshape  OutputDimensionality=Column vector (2-D)
  Reshape5 : Reshape  OutputDimensionality=Column vector (2-D)
  Reshape6 : Reshape  OutputDimensionality=Column vector (2-D)
  Vector Concatenate1 : Concatenate  NumInputs=3  Mode=Multidimensional array  ConcatenateDimension=2
  Q_sun_sun : Outport  VectorParamsAs1DForOutWhenUnconnected=off
  R_ss_2_i : Outport  Port=2  VectorParamsAs1DForOutWhenUnconnected=off
  wires:
  Direction Cosine Matrix to Quaternions1/1 -> Quaternion Inverse1/1
  Reshape4/1 -> Vector Concatenate1/2
  Dot Product1/1 -> Product1/1
  Sun_ECI/1 -> Normalization3/1
  Quaternion Inverse1/1 -> Q_sun_sun/1
  <VxVyVz_ECI>/1 -> Dot Product1/1, Plus1/1
  Plus1/1 -> Normalization4/1  "V-(V.z)z"
  Reshape6/1 -> Cross Product1/1, Vector Concatenate1/3
  Normalization3/1 -> Dot Product1/2, Product1/2, Reshape6/1  "z"
  Reshape5/1 -> Cross Product1/2, Vector Concatenate1/1
  Cross Product1/1 -> Reshape4/1  "y"
  Normalization4/1 -> Reshape5/1  "x"
  Product1/1 -> Plus1/2
  Vector Concatenate1/1 -> Reshape/1, Direction Cosine Matrix to Quaternions1/1
  Reshape/1 -> R_ss_2_i/1

== system distmodel_v4/Disturbance Torques /Aerodynamic Model/Calculate - Az & El Angle ==
  attitude : Inport
  Wind unit ECI : Inport  Port=2
  Atan2 : Trigonometry  Operator=atan2
  Constant1 : Constant  Value=2*pi
  Demux : Demux  Outputs=3
  Rotation : Product  Multiplication=Matrix(*)  RndMeth=Zero
  Scope3 : Scope
  Scope4 : Scope
  Sum : Sum  Inputs=|++
  Switch : Switch
  Trigonometric Function2 : Trigonometry  Operator=asin
  El : Outport
  Az : Outport  Port=2
  wires:
  attitude/1 -> Rotation/1  "ECI to BRF"
  Wind unit ECI/1 -> Rotation/2
  Rotation/1 -> Demux/1  "wind BRF"
  Demux/3 -> Trigonometric Function2/1
  Trigonometric Function2/1 -> El/1  "Elevation"
  Demux/1 -> Scope3/1, Atan2/2
  Demux/2 -> Atan2/1, Scope4/1
  Atan2/1 -> Switch/1, Switch/2, Sum/2
  Switch/1 -> Az/1
  Constant1/1 -> Sum/1
  Sum/1 -> Switch/3

== system distmodel_v4/Disturbance Torques /Aerodynamic Model/torque unit vector ==
  wind vector : Inport
  +x axis : Inport  Port=2
  Cross Product : vrlib/Utilities/Cross Product
  Display : Display
  Display1 : Display
  Normalize Vector : vrlib/Utilities/Normalize Vector  maxzero=0
  Scope1 : Scope  NumInputPorts=2
  Scope2 : Scope  NumInputPorts=2
  torque unit vector : Outport
  wires:
  Cross Product/1 -> Scope1/1, Normalize Vector/1
  wind vector/1 -> Display/1, Scope2/1, Cross Product/1
  +x axis/1 -> Display1/1, Scope2/2, Cross Product/2
  Normalize Vector/1 -> torque unit vector/1

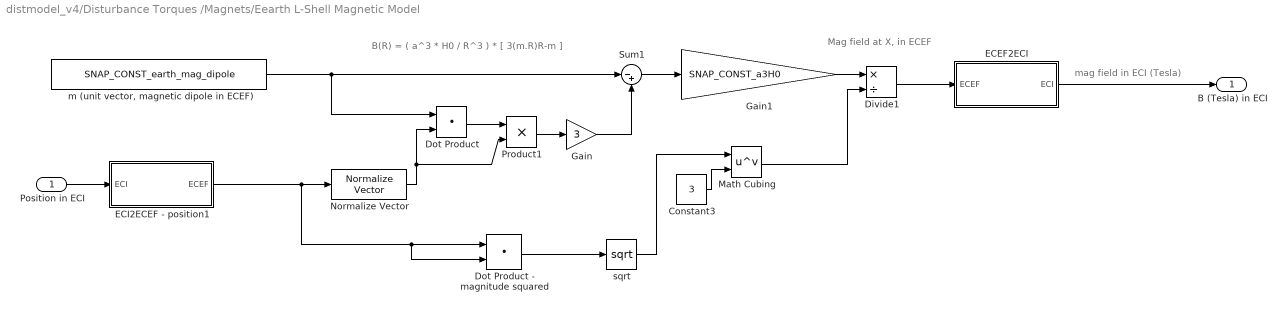
== system distmodel_v4/Disturbance Torques /Magnets/Eearth L-Shell Magnetic Model ==
  note: B(R) = ( a^3 * H0 / R^3 ) * [ 3(m.R)R-m ]
  note: Mag field at X, in ECEF
  note: mag field in ECI (Tesla)
  Position in ECI : Inport
  Constant3 : Constant  Value=3
  Divide1 : Product  Inputs=*/
  Dot Product : DotProduct  InputSameDT=on  OutDataTypeStr=Inherit: Inherit via internal rule
  Dot Product - magnitude squared : DotProduct  InputSameDT=on  OutDataTypeStr=Inherit: Inherit via internal rule
  ECEF2ECI : Subsystem
  ECI2ECEF - position1 : Subsystem
  Gain : Gain  Gain=3
  Gain1 : Gain  Gain=SNAP_CONST_a3H0
  Math Cubing : Math  Operator=pow  SignedPower=on  SaturateOnIntegerOverflow=on
  Normalize Vector : vrlib/Utilities/Normalize Vector  maxzero=0
  Product1 : Product  RndMeth=Zero
  Sum1 : Sum  Inputs=|-+
  "m (unit vector, magnetic dipole in ECEF)" : Constant  Value=SNAP_CONST_earth_mag_dipole
  sqrt : Math  Operator=sqrt  SignedPower=on  SaturateOnIntegerOverflow=on
  B (Tesla) in ECI : Outport
  wires:
  "m (unit vector, magnetic dipole in ECEF)"/1 -> Dot Product/1, Sum1/1
  ECI2ECEF - position1/1(ECEF) -> Dot Product - magnitude squared/2, Dot Product - magnitude squared/1, Normalize Vector/1
  Dot Product/1 -> Product1/1
  Product1/1 -> Gain/1
  Gain/1 -> Sum1/2
  Sum1/1 -> Gain1/1
  Gain1/1 -> Divide1/1
  Dot Product - magnitude squared/1 -> sqrt/1
  sqrt/1 -> Math Cubing/1
  Constant3/1 -> Math Cubing/2
  Math Cubing/1 -> Divide1/2
  Divide1/1 -> ECEF2ECI/1(ECEF)
  Normalize Vector/1 -> Dot Product/2, Product1/2
  ECEF2ECI/1(ECI) -> B (Tesla) in ECI/1
  Position in ECI/1 -> ECI2ECEF - position1/1(ECI)

== system distmodel_v4/Disturbance Torques /Magnets/Eearth L-Shell Magnetic Model/ECEF2ECI ==
  ECEF : Inport
  Constant1 : Constant  Value=[0 0]
  Constant3 : Constant  Value=SNAP_starting_ECI2ECEF_dcm
  Gain1 : Gain  Gain=-1
  Math Function2 : Math  Operator=transpose  SignedPower=on  SaturateOnIntegerOverflow=on
  Mux1 : Mux  Inputs=2
  Ramp2 : simulink/Sources/Ramp  slope="7.292115856e-5   %2*pi/(24*60*60)  %radians/second (one rotation per day )"  start=0  X0=0
  Rotation Angles to Direction Cosine Matrix1 : aerolibtransform2/Rotation Angles to Direction Cosine Matrix  rotationOrder=ZYX
      settings: SourceProductBaseCode=AE
  product 2 : Product  Multiplication=Matrix(*)  RndMeth=Zero
  product 4 : Product  Multiplication=Matrix(*)  RndMeth=Zero
  ECI : Outport
  wires:
  ECEF/1 -> product 4/1
  Ramp2/1 -> Gain1/1
  Gain1/1 -> Mux1/1
  Mux1/1 -> Rotation Angles to Direction Cosine Matrix1/1
  Constant1/1 -> Mux1/2
  product 2/1 -> Math Function2/1
  Rotation Angles to Direction Cosine Matrix1/1 -> product 2/2
  Constant3/1 -> product 2/1
  Math Function2/1 -> product 4/2
  product 4/1 -> ECI/1

== system distmodel_v4/Disturbance Torques /Magnets/Eearth L-Shell Magnetic Model/ECI2ECEF - position1 ==
  ECI : Inport
  Constant : Constant  Value=[0 0]
  Constant2 : Constant  Value=SNAP_starting_ECI2ECEF_dcm
  Gain : Gain  Gain=-1
  Mux : Mux  Inputs=2
  Ramp1 : simulink/Sources/Ramp  slope="7.292115856e-5   %2*pi/(24*60*60)  %radians/second (one rotation per day )"  start=0  X0=0
  Rotation Angles to Direction Cosine Matrix : aerolibtransform2/Rotation Angles to Direction Cosine Matrix  rotationOrder=ZYX
      settings: SourceProductBaseCode=AE
  product 1 : Product  Multiplication=Matrix(*)  RndMeth=Zero
  product 2 : Product  Multiplication=Matrix(*)  RndMeth=Zero
  ECEF : Outport
  wires:
  product 2/1 -> ECEF/1
  ECI/1 -> product 2/1
  Ramp1/1 -> Gain/1
  Gain/1 -> Mux/1
  Mux/1 -> Rotation Angles to Direction Cosine Matrix/1
  Constant/1 -> Mux/2
  product 1/1 -> product 2/2
  Rotation Angles to Direction Cosine Matrix/1 -> product 1/2
  Constant2/1 -> product 1/1

== matlab function distmodel_v4/Time propagator/JD to UTC ==
  data: JD input; Time_UTC output
function Time_UTC = fcn(JD)
    coder.extrinsic('datetime','datevec');
    Time_UTC = [0,0,0,0,0,0];
Time_UTC =  datevec(datetime(JD,'convertfrom','juliandate'));

== matlab function distmodel_v4/Time propagator/MATLAB Function ==
  data: t input; Y output; DOY output; S output
function [Y, DOY, S] = DOY(t)
Y = 2022 + fix(t/31557600);
DOY = 1+fix((t-floor(t/31557600)*31557600)/86400);
S = t - fix(t/31557600)*31557600 - (DOY-1)*86400;

== matlab function distmodel_v4/Time propagator/UTC to JD ==
  data: Time_UTC input; JD output
function JD = fcn(Time_UTC)

% JD = juliandate(Time_UTC);
JD = Dt2jD(Time_UTC);
